simulink model "sensors"  (R2018a)
settings: Solver=VariableStepAuto  StartTime=0.0  StopTime=10.0  RelTol=1e-3
undefined symbols (not defined in the file): ntc10k
libraries: fl_lib x4
settings Model: Creator=ChLan  LastModifiedBy=ChLan

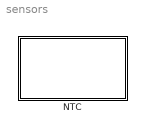
== system sensors ==
  NTC : Subsystem  mask{res_table=ntc10k}
      mask prompts: res_table "T-R Table"

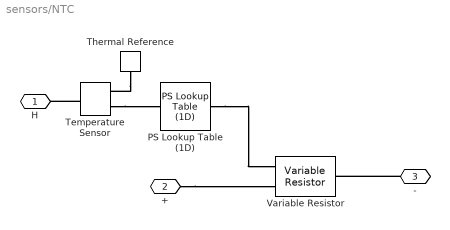
== system sensors/NTC ==
  PS Lookup Table (1D) : fl_lib/Physical Signals/Lookup Tables/PS Lookup Table (1D)  x=res_table(:,1) + 273.2  f=res_table(:,2)  interp_method=simscape.enum.interpolation.linear  extrap_method=simscape.enum.extrapolation.linear
      settings: SourceProductName=Simscape  SourceProductBaseCode=SS
  Temperature Sensor : fl_lib/Thermal/Thermal Sensors/Temperature Sensor
  Thermal Reference : fl_lib/Thermal/Thermal Elements/Thermal Reference
  Variable Resistor : fl_lib/Electrical/Electrical Elements/Variable Resistor  Rmin=0 Ohm  i_specify=off  i_priority=None  i=0 A  i_nominal_specify=off  i_nominal_unit=A  i_nominal_value=1  v_specify=off  v_priority=None  v=0 V  v_nominal_specify=off  v_nominal_unit=V  v_nominal_value=1
  H : PMIOPort  Side=Left
  + : PMIOPort  Port=2  Side=Left
  - : PMIOPort  Port=3  Side=Right
  connections:
  PS Lookup Table (1D)/RConn1 -- Variable Resistor/LConn1
  Temperature Sensor/RConn2 -- PS Lookup Table (1D)/LConn1
  +/RConn1 -- Variable Resistor/LConn2
  Temperature Sensor/LConn1 -- H/RConn1
  Thermal Reference/LConn1 -- Temperature Sensor/RConn1
  -/RConn1 -- Variable Resistor/RConn1
